simulink model "TestPuma560"  (R2018a)
settings: Solver=ode3  StartTime=0.0  StopTime=inf  FixedStep=0.001  MaxStep=0.01  RelTol=1e-3
PreLoadFcn:
  | %puma560=importrobot('puma560.urdf');
InitFcn:
  | %% Floor
  | YBT_Par.Floor.r = 54.5e-2; % m
  | YBT_Par.Floor.d = 1e-2;    % m
  | 
  | %% Cube and Fixed Payload
  | % Cube that moves on belt
  | YBT_Par.Cube.d = 3e-2;                         % m
  | YBT_Par.Cube.Con.rSph = YBT_Par.Cube.d*5e-2;   % m
  | YBT_Par.Cube.init_z = 1e-1; % m Lower surface above floor
  | YBT_Par.Cube.init_y = 40e-2+20e-2;             % m CG to World
  | YBT_Par.Cube.mark.base = YBT_Par.Cube.d*0.4;   % m
  | YBT_Par.Cube.mark.height = YBT_Par.Cube.d*0.7; % m
  | YBT_Par.Cube.mark.extrusion = [...
  |     YBT_Par.Cube.mark.base/2 -YBT_Par.Cube.mark.height/2;...
  |     YBT_Par.Cube.mark.base*0  YBT_Par.Cube.mark.height/2;...
  |    -YBT_Par.Cube.mark.base/2 -YBT_Par.Cube.mark.height/2]; %m
  | YBT_Par.Cube.mark.color = [0.0 0.3 0.5];       % RGB
model workspace (MAT data in the model file):
  color : struct (value not decoded)
  density : struct (value not decoded)
  floor : struct (value not decoded)
  motion_tc = 0.02
  robot : struct (value not decoded)
  workpiece : struct (value not decoded)
undefined symbols (not defined in the file): cube_d, X, Y, Z
libraries: sm_lib x88, fl_lib x17, nesl_utility x13, simulink x10, Contact_Forces_Lib x4
(part 3 of 3)

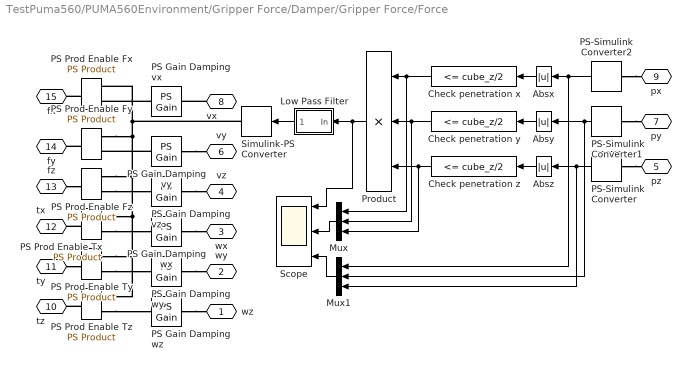
== system TestPuma560/PUMA560Environment/Gripper Force/Damper/Gripper Force/Force ==
  Absx : Abs  ZeroCross=off
  Absy : Abs  ZeroCross=off
  Absz : Abs  ZeroCross=off
  Check penetration x : simulink/Logic and Bit Operations/Compare To Constant  relop=<=  const=cube_z/2  OutDataTypeStr=boolean  ZeroCross=off
  Check penetration y : simulink/Logic and Bit Operations/Compare To Constant  relop=<=  const=cube_z/2  OutDataTypeStr=boolean  ZeroCross=off
  Check penetration z : simulink/Logic and Bit Operations/Compare To Constant  relop=<=  const=cube_z/2  OutDataTypeStr=boolean  ZeroCross=off
  Low Pass Filter : Subsystem  mask(First-order lag supporting vector signals){b=lpfilt_const_force, x_initial=0}
      mask prompts: b "Filter time constant"; x_initial "Initial output"
      mask help: Models a lag of the form 1/(b*s+1) where s is the Laplace operator.
  Mux : Mux  Inputs=3
  Mux1 : Mux  Inputs=3
  PS Gain Damping vx : fl_lib/Physical Signals/Functions/PS Gain  gain=-contact_b
  PS Gain Damping vy : fl_lib/Physical Signals/Functions/PS Gain  gain=-contact_b
  PS Gain Damping vz : fl_lib/Physical Signals/Functions/PS Gain  gain=-contact_b
  PS Gain Damping wx : fl_lib/Physical Signals/Functions/PS Gain  gain=-contact_b
  PS Gain Damping wy : fl_lib/Physical Signals/Functions/PS Gain  gain=-contact_b
  PS Gain Damping wz : fl_lib/Physical Signals/Functions/PS Gain  gain=-contact_b
  PS Prod Enable Fx : fl_lib/Physical Signals/Functions/PS Product
      settings: SourceProductName=Simscape
  PS Prod Enable Fy : fl_lib/Physical Signals/Functions/PS Product
      settings: SourceProductName=Simscape
  PS Prod Enable Fz : fl_lib/Physical Signals/Functions/PS Product
      settings: SourceProductName=Simscape
  PS Prod Enable Tx : fl_lib/Physical Signals/Functions/PS Product
      settings: SourceProductName=Simscape
  PS Prod Enable Ty : fl_lib/Physical Signals/Functions/PS Product
      settings: SourceProductName=Simscape
  PS Prod Enable Tz : fl_lib/Physical Signals/Functions/PS Product
      settings: SourceProductName=Simscape
  PS-Simulink Converter : nesl_utility/PS-Simulink Converter  PhysicalDomain=network_engine_domain  SubClassName=ps_output  LeftPortType=input  RightPortType=output  PseudoPeriodic=off  Frequencies=[]  Unit=1  AffineConversion=off
  PS-Simulink Converter1 : nesl_utility/PS-Simulink Converter  PhysicalDomain=network_engine_domain  SubClassName=ps_output  LeftPortType=input  RightPortType=output  PseudoPeriodic=off  Frequencies=[]  Unit=1  AffineConversion=off
  PS-Simulink Converter2 : nesl_utility/PS-Simulink Converter  PhysicalDomain=network_engine_domain  SubClassName=ps_output  LeftPortType=input  RightPortType=output  PseudoPeriodic=off  Frequencies=[]  Unit=1  AffineConversion=off
  Product : Product  Inputs=3  OutDataTypeStr=double
  Scope : Scope  NumInputPorts=3
  Simulink-PS Converter : nesl_utility/Simulink-PS Converter  PhysicalDomain=network_engine_domain  SubClassName=ps_input  LeftPortType=input  RightPortType=output  PseudoPeriodic=off  Frequencies=[]  NoiseDistribution=none  NoiseParameters=[]  Unit=1  AffineConversion=off  FilteringAndDerivatives=zero  SimscapeFilterOrder=1  InputFilterTimeConstant=0.001  UdotUserProvided=1
  wz : PMIOPort  Side=Left
  wy : PMIOPort  Port=2  Side=Left
  wx : PMIOPort  Port=3  Side=Left
  vz : PMIOPort  Port=4  Side=Left
  pz : PMIOPort  Port=5  Side=Left
  vy : PMIOPort  Port=6  Side=Left
  py : PMIOPort  Port=7  Side=Left
  vx : PMIOPort  Port=8  Side=Left
  px : PMIOPort  Port=9  Side=Left
  tz : PMIOPort  Port=10  Side=Right
  ty : PMIOPort  Port=11  Side=Right
  tx : PMIOPort  Port=12  Side=Right
  fz : PMIOPort  Port=13  Side=Right
  fy : PMIOPort  Port=14  Side=Right
  fx : PMIOPort  Port=15  Side=Right
  wires:
  PS-Simulink Converter1/1 -> Absy/1, Mux1/2
  PS-Simulink Converter2/1 -> Mux1/1, Absx/1
  Check penetration x/1 -> Mux/1, Product/1
  Check penetration y/1 -> Mux/2, Product/2
  Check penetration z/1 -> Mux/3, Product/3
  Mux/1 -> Scope/2
  Mux1/1 -> Scope/3
  PS-Simulink Converter/1 -> Mux1/3, Absz/1
  Absx/1 -> Check penetration x/1
  Absy/1 -> Check penetration y/1
  Absz/1 -> Check penetration z/1
  Product/1 -> Scope/1, Low Pass Filter/1(In)
  Low Pass Filter/1(Out) -> Simulink-PS Converter/1
  connections:
  vx/RConn1 -- PS Gain Damping vx/LConn1
  PS Gain Damping vx/RConn1 -- PS Prod Enable Fx/LConn2
  PS Gain Damping vy/RConn1 -- PS Prod Enable Fy/LConn2
  PS Gain Damping vy/LConn1 -- vy/RConn1
  PS Gain Damping vz/LConn1 -- vz/RConn1
  PS Prod Enable Fz/LConn2 -- PS Gain Damping vz/RConn1
  PS Prod Enable Tx/LConn2 -- PS Gain Damping wx/RConn1
  PS Gain Damping wx/LConn1 -- wx/RConn1
  PS Prod Enable Ty/LConn2 -- PS Gain Damping wy/RConn1
  PS Gain Damping wy/LConn1 -- wy/RConn1
  PS Prod Enable Tz/LConn2 -- PS Gain Damping wz/RConn1
  PS Gain Damping wz/LConn1 -- wz/RConn1
  PS-Simulink Converter/LConn1 -- pz/RConn1
  PS-Simulink Converter1/LConn1 -- py/RConn1
  PS-Simulink Converter2/LConn1 -- px/RConn1
  PS Prod Enable Tx/LConn1 -- PS Prod Enable Tz/LConn1 -- PS Prod Enable Ty/LConn1 -- PS Prod Enable Fz/LConn1 -- PS Prod Enable Fy/LConn1 -- PS Prod Enable Fx/LConn1 -- Simulink-PS Converter/RConn1
  PS Prod Enable Fx/RConn1 -- fx/RConn1
  PS Prod Enable Tz/RConn1 -- tz/RConn1
  ty/RConn1 -- PS Prod Enable Ty/RConn1
  PS Prod Enable Tx/RConn1 -- tx/RConn1
  fz/RConn1 -- PS Prod Enable Fz/RConn1
  PS Prod Enable Fy/RConn1 -- fy/RConn1

== system TestPuma560/PUMA560Environment/Gripper Force/Damper/Gripper Force/Relative vz ==
  Fingers : Subsystem  VariantControl=Fingers
  Housing : Subsystem  VariantControl=Housing
  vz fa : PMIOPort  Side=Left
  Box : PMIOPort  Port=2  Side=Left
  b : PMIOPort  Port=3  Side=Left
  E : PMIOPort  Port=4  Side=Left
  vz : PMIOPort  Port=5  Side=Right

== system TestPuma560/PUMA560Environment/Gripper Force/Damper/Gripper Force/Force/Low Pass Filter ==
  In : Inport
  Gain : Gain  Gain=1./b
  Integrator : Integrator  InitialCondition=x_initial.*b
  Sum : Sum  Inputs=|+-  SaturateOnIntegerOverflow=on  InputSameDT=on  OutDataTypeStr=Inherit: Same as first input
  Out : Outport
  wires:
  Sum/1 -> Integrator/1
  In/1 -> Sum/1
  Integrator/1 -> Gain/1
  Gain/1 -> Sum/2, Out/1

== system TestPuma560/PUMA560Environment/Gripper Force/Damper/Gripper Force/Relative vz/Fingers ==
  PS Gain : fl_lib/Physical Signals/Functions/PS Gain  gain=1
  PS Gain1 : fl_lib/Physical Signals/Functions/PS Gain  gain=1
  PS Subtract : fl_lib/Physical Signals/Functions/PS Subtract
      settings: SourceProductName=Simscape
  Transform Sensor : sm_lib/Frames and Transforms/Transform Sensor  MeasurementFrame=Base  SenseAngle=off  SenseAxis=off  SenseAngle1=off  SenseAngle2=off  SenseAngle3=off  SenseQ=off  SenseR=off  SenseOmegaX=off  SenseOmegaY=off  SenseOmegaZ=off  SenseOmega1=off  SenseOmega2=off  SenseOmega3=off  SenseQDot=off  SenseRDot=off  SenseAlphaX=off  SenseAlphaY=off  SenseAlphaZ=off  SenseAlpha1=off  SenseAlpha2=off  SenseAlpha3=off  SenseQDDot=off  SenseRDDot=off  SenseX=off  SenseY=off  SenseZ=off  SenseRad=off  SenseAzim=off  SenseDist=off  SenseInc=off  SenseXDot=off  SenseYDot=off  SenseZDot=on  SenseRadDot=off  SenseAzimDot=off  SenseDistDot=off  SenseIncDot=off  SenseXDDot=off  SenseYDDot=off  SenseZDDot=off  SenseRadDDot=off  SenseAzimDDot=off  SenseDistDDot=off  SenseIncDDot=off
  vz fa : PMIOPort  Side=Left
  Box : PMIOPort  Port=2  Side=Left
  b : PMIOPort  Port=3  Side=Left
  E : PMIOPort  Port=4  Side=Left
  vz : PMIOPort  Port=5  Side=Right
  connections:
  PS Subtract/LConn1 -- vz fa/RConn1
  PS Gain/LConn1 -- Transform Sensor/RConn2
  Transform Sensor/LConn1 -- b/RConn1
  PS Subtract/RConn1 -- PS Gain1/LConn1
  PS Gain/RConn1 -- PS Subtract/LConn2
  Transform Sensor/RConn1 -- Box/RConn1
  PS Gain1/RConn1 -- vz/RConn1

== system TestPuma560/PUMA560Environment/Gripper Force/Damper/Gripper Force/Relative vz/Housing ==
  PS Gain : fl_lib/Physical Signals/Functions/PS Gain  gain=1
  PS Terminator : fl_lib/Physical Signals/Sinks/PS Terminator
      settings: SourceProductName=Simscape
  Transform Sensor : sm_lib/Frames and Transforms/Transform Sensor  MeasurementFrame=Base  SenseAngle=off  SenseAxis=off  SenseAngle1=off  SenseAngle2=off  SenseAngle3=off  SenseQ=off  SenseR=off  SenseOmegaX=off  SenseOmegaY=off  SenseOmegaZ=off  SenseOmega1=off  SenseOmega2=off  SenseOmega3=off  SenseQDot=off  SenseRDot=off  SenseAlphaX=off  SenseAlphaY=off  SenseAlphaZ=off  SenseAlpha1=off  SenseAlpha2=off  SenseAlpha3=off  SenseQDDot=off  SenseRDDot=off  SenseX=off  SenseY=off  SenseZ=off  SenseRad=off  SenseAzim=off  SenseDist=off  SenseInc=off  SenseXDot=off  SenseYDot=off  SenseZDot=on  SenseRadDot=off  SenseAzimDot=off  SenseDistDot=off  SenseIncDot=off  SenseXDDot=off  SenseYDDot=off  SenseZDDot=off  SenseRadDDot=off  SenseAzimDDot=off  SenseDistDDot=off  SenseIncDDot=off
  vz fa : PMIOPort  Side=Left
  Box : PMIOPort  Port=2  Side=Left
  b : PMIOPort  Port=3  Side=Left
  E : PMIOPort  Port=4  Side=Left
  vz : PMIOPort  Port=5  Side=Right
  connections:
  Transform Sensor/RConn1 -- Box/RConn1
  PS Gain/RConn1 -- vz/RConn1
  Transform Sensor/LConn1 -- E/RConn1
  PS Gain/LConn1 -- Transform Sensor/RConn2
  PS Terminator/LConn1 -- vz fa/RConn1

== matlab function TestPuma560/MATLAB Function1 ==
  data: Pos input double; AllSloverTheta output; Rotation input double
function AllSloverTheta =InverseSolver_MDH(Pos,Rotation)
%#codegen
%% coder.extrinsic 声明外部函数。
%% 在仿真期间，代码生成器会为外部函数的调用生成代码，但不会生成函数的内部代码。
coder.extrinsic('disp');
%% 建立机器人DH参数，初始状态为竖直状态
%% L1=Link('d',144,'a',0,'alpha',0,'modified'); 
%% L2=Link('d',0,'a',0,'alpha',pi/2,'offset',-pi/2,'modified');
%% L3=Link('d',0,'a',-264,'alpha',0,'modified');
%% L4=Link('d',106,'a',-236,'alpha',0,'offset',-pi/2,'modified');
%% L5=Link('d',114,'a',0,'alpha',pi/2,'modified');
%% L6=Link('d',67,'a',0,'alpha',-pi/2,'modified');
    AllSloverTheta = zeros(8,6);A=zeros(1,4);
 %%            [alpha, a,     d,  offset] 
           DH_JXB =[0     0          0      0; 
                    90    0          0      0;
                    0     0.4318  0.1501    0; 
                   -90    0.203   0.4318    0; 
                    90    0          0      0; 
                   -90    0          0      0];
   % *****************************************************************************            
    p2=DH_JXB(2,4);p4=DH_JXB(4,4);
    a2=DH_JXB(3,2);a3=DH_JXB(4,2);d1=DH_JXB(1,3);d4=DH_JXB(4,3);d5=DH_JXB(5,3);
    X=Pos(1,1);Y=Pos(1,2);Z=Pos(1,3);
    gama=Rotation(1,1)*pi/180;beta=Rotation(1,2)*pi/180;alpha=Rotation(1,3)*pi/180;
    theta7=0;a6=0;afa6=0;d7=DH_JXB(6,3);
    % *****************************************************************************
    T67=[   cos(theta7),-sin(theta7),0,a6;
                sin(theta7)*cos(afa6),cos(theta7)*cos(afa6),-sin(afa6),-sin(afa6)*d7;
                sin(theta7)*sin(afa6),cos(theta7)*sin(afa6),cos(afa6),cos(afa6)*d7;
                0,0,0,1
             ];
   T_goat=[  cos(beta)*cos(gama),-cos(beta)*sin(gama),sin(beta),X;
                   sin(alpha)*sin(beta)*cos(gama)+cos(alpha)*sin(gama), -sin(alpha)*sin(beta)*sin(gama)+cos(alpha)*cos(gama), -sin(alpha)*cos(beta),Y;
                  -cos(alpha)*sin(beta)*cos(gama)+sin(alpha)*sin(gama), cos(alpha)*sin(beta)*sin(gama)+sin(alpha)*cos(gama),  cos(alpha)*cos(beta),Z;
                  0,0,0,1
              ];
    T06=T_goat/T67;
    
    nx=T06(1,1);ny=T06(2,1);
    ox=T06(1,2);oy=T06(2,2);
    ax=T06(1,3);ay=T06(2,3);az=T06(3,3);
    % X-Y-Z
    px=T06(1,4);py=T06(2,4);pz=T06(3,4);
    
    k=0;
    ForJudgment=px^2+py^2-d4^2;
    
    if ForJudgment<-1e-6
        disp('Out of workspace Unable to solve');
    else      
        if ForJudgment>=-1e-6&&ForJudgment<0
            ForJudgment=0;
        end
        theta1_1=atan2(py,px)-atan2(-d4,sqrt(ForJudgment));
        theta1_2=atan2(py,px)-atan2(-d4,-sqrt(ForJudgment));
        
        S5_1=sqrt((-sin(theta1_1)*nx+cos(theta1_1)*ny)^2+(-sin(theta1_1)*ox+cos(theta1_1)*oy)^2);
        theta5_1=atan2(S5_1,sin(theta1_1)*ax-cos(theta1_1)*ay);
        S5_2=-sqrt((-sin(theta1_1)*nx+cos(theta1_1)*ny)^2+(-sin(theta1_1)*ox+cos(theta1_1)*oy)^2);
        theta5_2=atan2(S5_2,sin(theta1_1)*ax-cos(theta1_1)*ay);
        S5_3=sqrt((-sin(theta1_2)*nx+cos(theta1_2)*ny)^2+(-sin(theta1_2)*ox+cos(theta1_2)*oy)^2);
        theta5_3=atan2(S5_3,sin(theta1_2)*ax-cos(theta1_2)*ay);
        S5_4=-sqrt((-sin(theta1_2)*nx+cos(theta1_2)*ny)^2+(-sin(theta1_2)*ox+cos(theta1_2)*oy)^2);
        theta5_4=atan2(S5_4,sin(theta1_2)*ax-cos(theta1_2)*ay);
        
        S234 = [0; 0; 0; 0];C234 = [0; 0; 0; 0];
        B = [0; 0; 0; 0];B1 = [0; 0; 0; 0];B2 = [0; 0; 0; 0];
        C = [0; 0; 0; 0];
        theta2 = [0; 0; 0; 0; 0; 0; 0; 0];
        theta23 = [0; 0; 0; 0; 0; 0; 0; 0];
        theta234 = [0; 0; 0; 0; 0; 0; 0; 0];
        theta3 = [0; 0; 0; 0; 0; 0; 0; 0];
        theta4 = [0; 0; 0; 0; 0; 0; 0; 0];
        
        if abs(S5_1)>1e-6
            theta6_1=atan2((-sin(theta1_1)*ox+cos(theta1_1)*oy)/S5_1,(sin(theta1_1)*nx-cos(theta1_1)*ny)/S5_1);
            S234(1)=-az/S5_1;C234(1)=-(cos(theta1_1)*ax+sin(theta1_1)*ay)/S5_1;theta234(1)=atan2(S234(1),C234(1));
            B1(1)=cos(theta1_1)*px+sin(theta1_1)*py-d5*S234(1);B2(1)=pz-d1+d5*C234(1);A(1)=-2*B2(1)*a2;B(1)=2*B1(1)*a2;C(1)=B1(1)^2+B2(1)^2+a2^2-a3^2;
            if A(1)^2+B(1)^2-C(1)^2>=0
                theta2(1)=atan2(B(1),A(1))-atan2(C(1),sqrt(A(1)^2+B(1)^2-C(1)^2));
                theta2(2)=atan2(B(1),A(1))-atan2(C(1),-sqrt(A(1)^2+B(1)^2-C(1)^2));
                theta23(1)=atan2((B2(1)-a2*sin(theta2(1)))/a3,(B1(1)-a2*cos(theta2(1)))/a3);theta23(2)=atan2((B2(1)-a2*sin(theta2(2)))/a3,(B1(1)-a2*cos(theta2(2)))/a3);
                theta4(1)=theta234(1)-theta23(1);
                theta4(2)=theta234(1)-theta23(2);
                theta3(1)=theta23(1)-theta2(1);
                theta3(2)=theta23(2)-theta2(2);
                AllSloverTheta(k+1,:)=[theta1_1 theta2(1)-p2*pi/180 theta3(1) theta4(1)-p4*pi/180 theta5_1 theta6_1];
                AllSloverTheta(k+2,:)=[theta1_1 theta2(2)-p2*pi/180 theta3(2) theta4(2)-p4*pi/180 theta5_1 theta6_1];
                k=k+2;
            end
        end
        if abs(S5_2)>1e-6
            theta6_2=atan2((-sin(theta1_1)*ox+cos(theta1_1)*oy)/S5_2,(sin(theta1_1)*nx-cos(theta1_1)*ny)/S5_2);
            S234(2)=-az/S5_2;C234(2)=-(cos(theta1_1)*ax+sin(theta1_1)*ay)/S5_2;theta234(2)=atan2(S234(2),C234(2));
            B1(2)=cos(theta1_1)*px+sin(theta1_1)*py-d5*S234(2);B2(2)=pz-d1+d5*C234(2);A(2)=-2*B2(2)*a2;B(2)=2*B1(2)*a2;C(2)=B1(2)^2+B2(2)^2+a2^2-a3^2;
            if A(2)^2+B(2)^2-C(2)^2>=0
                theta2(3)=atan2(B(2),A(2))-atan2(C(2),sqrt(A(2)^2+B(2)^2-C(2)^2));
                theta2(4)=atan2(B(2),A(2))-atan2(C(2),-sqrt(A(2)^2+B(2)^2-C(2)^2));
                theta23(3)=atan2((B2(2)-a2*sin(theta2(3)))/a3,(B1(2)-a2*cos(theta2(3)))/a3);theta23(4)=atan2((B2(2)-a2*sin(theta2(4)))/a3,(B1(2)-a2*cos(theta2(4)))/a3);
                theta4(3)=theta234(2)-theta23(3);
                theta4(4)=theta234(2)-theta23(4);
                theta3(3)=theta23(3)-theta2(3);
                theta3(4)=theta23(4)-theta2(4);
                AllSloverTheta(k+1,:)=[theta1_1 theta2(3)-p2*pi/180 theta3(3) theta4(3)-p4*pi/180 theta5_2 theta6_2];
                AllSloverTheta(k+2,:)=[theta1_1 theta2(4)-p2*pi/180 theta3(4) theta4(4)-p4*pi/180 theta5_2 theta6_2];
                k=k+2;
            end
        end
        if abs(S5_3)>1e-6
            theta6_3=atan2((-sin(theta1_2)*ox+cos(theta1_2)*oy)/S5_3,(sin(theta1_2)*nx-cos(theta1_2)*ny)/S5_3);
            S234(3)=-az/S5_3;C234(3)=-(cos(theta1_2)*ax+sin(theta1_2)*ay)/S5_3;theta234(3)=atan2(S234(3),C234(3));
            B1(3)=cos(theta1_2)*px+sin(theta1_2)*py-d5*S234(3);B2(3)=pz-d1+d5*C234(3);A(3)=-2*B2(3)*a2;B(3)=2*B1(3)*a2;C(3)=B1(3)^2+B2(3)^2+a2^2-a3^2;
            if A(3)^2+B(3)^2-C(3)^2>=0
                theta2(5)=atan2(B(3),A(3))-atan2(C(3),sqrt(A(3)^2+B(3)^2-C(3)^2));
                theta2(6)=atan2(B(3),A(3))-atan2(C(3),-sqrt(A(3)^2+B(3)^2-C(3)^2));
                theta23(5)=atan2((B2(3)-a2*sin(theta2(5)))/a3,(B1(3)-a2*cos(theta2(5)))/a3);theta23(6)=atan2((B2(3)-a2*sin(theta2(6)))/a3,(B1(3)-a2*cos(theta2(6)))/a3);
                theta4(5)=theta234(3)-theta23(5);
                theta4(6)=theta234(3)-theta23(6);
                theta3(5)=theta23(5)-theta2(5);
                theta3(6)=theta23(6)-theta2(6);
                AllSloverTheta(k+1,:)=[theta1_2 theta2(5)-p2*pi/180 theta3(5) theta4(5)-p4*pi/180 theta5_3 theta6_3];
                AllSloverTheta(k+2,:)=[theta1_2 theta2(6)-p2*pi/180 theta3(6) theta4(6)-p4*pi/180 theta5_3 theta6_3];
                k=k+2;
            end
        end
        if abs(S5_4)>1e-6
            theta6_4=atan2((-sin(theta1_2)*ox+cos(theta1_2)*oy)/S5_4,(sin(theta1_2)*nx-cos(theta1_2)*ny)/S5_4);
            S234(4)=-az/S5_4;C234(4)=-(cos(theta1_2)*ax+sin(theta1_2)*ay)/S5_4;theta234(4)=atan2(S234(4),C234(4));
            B1(4)=cos(theta1_2)*px+sin(theta1_2)*py-d5*S234(4);B2(4)=pz-d1+d5*C234(4);A(4)=-2*B2(4)*a2;B(4)=2*B1(4)*a2;C(4)=B1(4)^2+B2(4)^2+a2^2-a3^2;
            if A(4)^2+B(4)^2-C(4)^2>=0
                theta2(7)=atan2(B(4),A(4))-atan2(C(4),sqrt(A(4)^2+B(4)^2-C(4)^2));
                theta2(8)=atan2(B(4),A(4))-atan2(C(4),-sqrt(A(4)^2+B(4)^2-C(4)^2));
                theta23(7)=atan2((B2(4)-a2*sin(theta2(7)))/a3,(B1(4)-a2*cos(theta2(7)))/a3);theta23(8)=atan2((B2(4)-a2*sin(theta2(8)))/a3,(B1(4)-a2*cos(theta2(8)))/a3);
                theta4(7)=theta234(4)-theta23(7);
                theta4(8)=theta234(4)-theta23(8);
                theta3(7)=theta23(7)-theta2(7);
                theta3(8)=theta23(8)-theta2(8);
                AllSloverTheta(k+1,:)=[theta1_2 theta2(7)-p2*pi/180 theta3(7) theta4(7)-p4*pi/180 theta5_4 theta6_4];
                AllSloverTheta(k+2,:)=[theta1_2 theta2(8)-p2*pi/180 theta3(8) theta4(8)-p4*pi/180 theta5_4 theta6_4];
                k=k+2;
            end
        end
        
        if k>0
            AllSloverTheta=AllSloverTheta*180/pi;%将弧度转化成角度
            for i=1:k
                for j=1:6
                    if AllSloverTheta(i,j)<=-180
                        AllSloverTheta(i,j)=AllSloverTheta(i,j)+360;%将角度限定在-180—+180
                    elseif AllSloverTheta(i,j)>180
                        AllSloverTheta(i,j)=AllSloverTheta(i,j)-360;%将角度限定在-180—+180
                    end
                end
            end
        else 
                disp('Singular position Unable to solve');
        end
    end
end

== matlab function TestPuma560/MATLAB Function ==
  data: theta input; Pos output; Rotation output double
%% MDH，PUMA560 Forward Kinematics Solver
function [Pos,Rotation]=PUMA560ForwardWay(theta)
% Initial the parameters
rpy=zeros(1,3);
        a2 = 0.4318;
        a3 = 0.0203;
        d3 = 0.1501;
        d4 = 0.4318;
t1=theta(1,1);t2=theta(2,1); t3=theta(3,1)-90; t4=theta(4,1); t5=theta(5,1); t6=theta(6,1);     
        T_01 = tmat(0, 0, 0, t1);
        T_12 = tmat(90, 0, 0, t2);
        T_23 = tmat(0, a2, d3, t3);
        T_34 = tmat(-90, a3, d4, t4);
        T_45 = tmat(90, 0, 0, t5);
        T_56 = tmat(-90, 0, 0, t6);

 % Each link fram to base frame transformation
        T_02 = T_01*T_12;
        T_03 = T_02*T_23;
        T_04 = T_03*T_34;
        T_05 = T_04*T_45;
        T_06 = T_05*T_56;
        
X=T_06(1,4);Y=T_06(2,4);Z=T_06(3,4);
R=T_06;
    if abs(abs(R(1,3)) - 1) < eps  % when |R13| == 1
        % singularity
        rpy(1) = 0;  % roll is zero
        if R(1,3) > 0
        rpy(3) = atan2( R(3,2), R(2,2));   % R+Y
        else
             rpy(3) = -atan2( R(2,1), R(3,1));   % R-Y
        end
        rpy(2) = asin(R(1,3));
    else
        rpy(1) = -atan2(R(1,2), R(1,1));
        rpy(3) = -atan2(R(2,3), R(3,3));

        rpy(2) = atan(R(1,3)*cos(rpy(1))/R(1,1));
    end
    RPY=rpy*180/pi;
    Rall=RPY(1);Pitch=RPY(2);Yaw=RPY(3);
    Pos=[X Y Z]; 
    Rotation=[Rall Pitch Yaw];
% The foremost transformation 
function T = tmat(alpha, a, d, theta)%改进DH方法，坐标变换过程看出Craig
        % tmat(alpha, a, d, theta) (T-Matrix used in Robotics)
        % The homogeneous transformation called the "T-MATRIX"
        % as used in the Kinematic Equations for robotic type
        % systems (or equivalent).
        %
        % This is equation 3.6 in Craig's "Introduction to Robotics."
        % alpha, a, d, theta are the Denavit-Hartenberg parameters.
        %
        % (NOTE: ALL ANGLES MUST BE IN DEGREES.)
        %
        alpha = alpha*pi/180;    %Note: alpha is in radians.
        theta = theta*pi/180;    %Note: theta is in radians.
        c = cos(theta);
        s = sin(theta);
        ca = cos(alpha);
        sa = sin(alpha);
        T = [c -s 0 a; s*ca c*ca -sa -sa*d; s*sa c*sa ca ca*d; 0 0 0 1];
end

end

== matlab function TestPuma560/MATLAB Function2 ==
  data: Pos input double; SloverTheta output; Rotation input double
 function SloverTheta  =InverseSolver_MDH(Pos,Rotation)
%#codegen
%% coder.extrinsic 声明外部函数。
%% 在仿真期间，代码生成器会为外部函数的调用生成代码，但不会生成函数的内部代码。
coder.extrinsic('disp');  
SloverTheta = zeros(1,6);
 %%            [alpha, a,     d,  offset] 
           DH_JXB =[0     0          0      0; 
                    90    0          0      0;
                    0     0.4318  0.1501    0; 
                   -90    0.203   0.4318    0; 
                    90    0          0      0; 
                   -90    0          0      0];
 % *****************************************************************************             
    p2=DH_JXB(2,4);p4=DH_JXB(4,4);
    a2=DH_JXB(3,2);a3=DH_JXB(4,2);d3=DH_JXB(1,3);d4=DH_JXB(4,3);d5=DH_JXB(5,3);
    Px=Pos(1,1);Py=Pos(1,2);Pz=Pos(1,3);
    gama=Rotation(1,1)*pi/180;beta=Rotation(1,2)*pi/180;alpha=Rotation(1,3)*pi/180;
    theta7=0;a6=0;afa6=0;d7=DH_JXB(6,3);
    T67=[   cos(theta7),-sin(theta7),0,a6;
                sin(theta7)*cos(afa6),cos(theta7)*cos(afa6),-sin(afa6),-sin(afa6)*d7;
                sin(theta7)*sin(afa6),cos(theta7)*sin(afa6),cos(afa6),cos(afa6)*d7;
                0,0,0,1
             ];
    T_goat=[  cos(beta)*cos(gama),-cos(beta)*sin(gama),sin(beta),Px;
                   sin(alpha)*sin(beta)*cos(gama)+cos(alpha)*sin(gama), -sin(alpha)*sin(beta)*sin(gama)+cos(alpha)*cos(gama), -sin(alpha)*cos(beta),Py;
                  -cos(alpha)*sin(beta)*cos(gama)+sin(alpha)*sin(gama), cos(alpha)*sin(beta)*sin(gama)+sin(alpha)*cos(gama),  cos(alpha)*cos(beta),Pz;
                  0,0,0,1
              ];
    T06=T_goat/T67;
    
r11=T06(1,1);r12=T06(1,2);r13=T06(1,3);
r21=T06(2,1);r22=T06(2,2);r23=T06(2,3);
r31=T06(3,1);r32=T06(3,2);r33=T06(3,3);
    % *****************************************************************************              
                %rho = sqrt(Px^2+Py^2);
                %phi = atan2(Py,Px);     % atan2 returns angles between 2pi,-2pi
                K = (Px^2+Py^2+Pz^2-a2^2-a3^2-d3^2-d4^2)/(2*a2);
                    
                theta1 = (atan2(Py,Px)-atan2(d3,sqrt(Px^2+Py^2-d3^2)));
                c1 = cos(theta1);
                s1 = sin(theta1);
          
                theta3 = (atan2(a3,d4)-atan2(real(K),real(sqrt(a3^2+d4^2-K^2))));
                c3 = cos(theta3);
                s3 = sin(theta3);

                t23 = atan2((-a3-a2*c3)*Pz-(c1*Px+s1*Py)*(d4-a2*s3),(a2*s3-d4)*Pz+(a3+a2*c3)*(c1*Px+s1*Py));
                theta2 = (t23 - theta3);
                c2 = cos(theta2);
                s2 = sin(theta2);
                s23 = ((-a3-a2*c3)*Pz+(c1*Px+s1*Py)*(a2*s3-d4))/(Pz^2+(c1*Px+s1*Py)^2);
                c23 = ((a2*s3-d4)*Pz+(a3+a2*c3)*(c1*Px+s1*Py))/(Pz^2+(c1*Px+s1*Py)^2);
                
                theta4 = atan2(-r13*s1+r23*c1,-r13*c1*c23-r23*s1*c23 + r33*s23);
                c4 = cos(theta4);
                s4 = sin (theta4);
                
                s5 = -(r13*(c1*c23*c4+s1*s4)+r23*(s1*c23*c4-c1*s4)-r33*(s23*c4));
                c5 = r13*(-c1*s23)+r23*(-s1*s23)+r33*(-c23);
                theta5 = atan2(s5,c5);

                s6 = -r11*(c1*c23*s4-s1*c4)-r21*(s1*c23*s4+c1*c4)+r31*(s23*s4);
                c6 = r11*((c1*c23*c4+s1*s4)*c5-c1*s23*s5)+r21*((s1*c23*c4-c1*s4)*c5-s1*s23*s5)-r31*(s23*c4*c5+c23*s5);
                theta6 = atan2(s6,c6);

                % From rad to deg
                theta1 = theta1*180/pi;
                theta2 = theta2*180/pi;
                theta3 = theta3*180/pi;
                theta4 = theta4*180/pi;
                theta5 = theta5*180/pi;
                theta6 = theta6*180/pi;
                SloverTheta=[theta1,theta2,theta3,theta4,theta5,theta6]
 end
